simulink model "Audio_Signal_Processing"  (R2020b)
settings: Solver=FixedStepDiscrete  StartTime=0.0  StopTime=10  RelTol=1e-3
libraries: dsparch4 x3, dspvision x1, audioeffects x1
settings Model: Creator=jferrari  LastModifiedBy=Jack
settings SolverCC: AutoInsertRateTranBlk=on
settings DataIOCC: LimitDataPoints=on  SaveOutput=off  SignalLogging=off  SaveTime=off
settings OptimizationCC: LifeSpan=inf
settings DebuggingCC: AlgebraicLoopMsg=error  SingleTaskRateTransMsg=error  AllowSymbolicDim=off  SFUnexpectedBacktrackingDiag=warning  SFNoUnconditionalDefaultTransitionDiag=warning  SFExecutionAtInitializationDiag=none  ArithmeticOperatorsInVariantConditions=warning
settings SFSimCC: SimUseLocalCustomCode=off  CustomCodeUndefinedFunction=UseInterfaceOnly
settings RTWCC: RTWUseLocalCustomCode=off
settings CodeAppCC: StateflowObjectComments=on
settings GRTTargetCC: TargetLangStandard=C89/C90 (ANSI)
settings ConfigComp: CovMetricSettings=dw  CovSaveCumulativeToWorkspaceVar=on  CovSaveSingleToWorkspaceVar=on  CovExternalEMLEnable=off  CovSFcnEnable=off

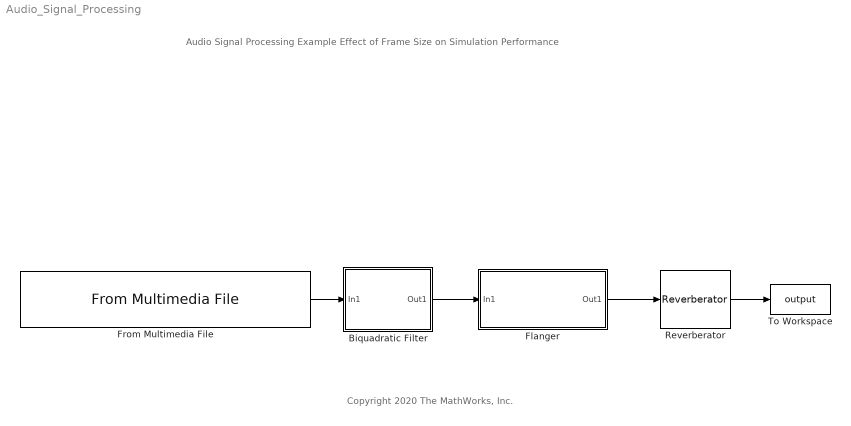
== system Audio_Signal_Processing ==
  note: Copyright 2020 The MathWorks, Inc.
  note: Audio Signal Processing Example
      | Effect of Frame Size on Simulation Performance
  Biquadratic Filter : Subsystem
  Flanger : Subsystem  mask(Flanger){Delay=0.001, Depth=30, Rate=0.25, FeedbackLevel=0.4, WetDryMix=0.5, SampleRate=44100}
      mask prompts: Delay "Base delay (s)"; Rate "Rate (Hz)"; FeedbackLevel "Feedback gain"; WetDryMix "Wet/dry mix"; SampleRate "Input sample rate (Hz):"
      mask help: Apply flanging effect on audio signal.
      mask Display: disp('Flanger')
  From Multimedia File : dspvision/From Multimedia File  inputFilename=/Users/Jack/OneDrive - MathWorks/Documents/Simulink/DSP Project/Frame-Based Processing Example/RockGuitar-16-44p1-stereo-10secs.mp3  readRange=[1 Inf]  loop=on  numPlays=1  outputStreams=Audio only  videoDataType=single  audioDataType=double  inheritSampleTime=on  userDefinedSampleTime=1/30  noAudioOutput=off  isIntensityVideo=off  fourcc=RGB  colorVideoFormat=Separate color signals  outputEOF=off  dataOrg=Column-major  audioFrameSize=1024  computeAudioFrameSize=off  outSamplingMode=Sample based
  Reverberator : audioeffects/Reverberator  PreDelayPort=off  PreDelay=0.0  HighCutFrequencyPort=off  HighCutFrequency=17003.0  DiffusionPort=off  Diffusion=0.0  DecayFactorPort=off  DecayFactor=0.790  HighFrequencyDampingPort=off  HighFrequencyDamping=0.0005  WetDryMixPort=off  WetDryMix=0.3  InheritSampleRate=on  SampleRate=44100  SimulateUsing=Interpreted execution
      settings: SourceProductBaseCode=AU
  To Workspace : ToWorkspace  VariableName=output  SampleTime=-1
      settings: Save2DSignal=2-D array (concatenate along first dimension)
  wires:
  From Multimedia File/1 -> Biquadratic Filter/1(In1)
  Reverberator/1 -> To Workspace/1
  Biquadratic Filter/1(Out1) -> Flanger/1(In1)
  Flanger/1(Out1) -> Reverberator/1

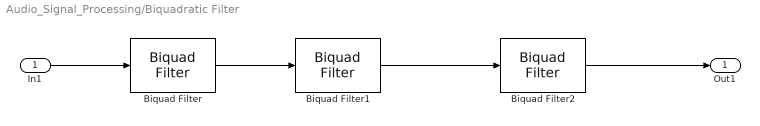
== system Audio_Signal_Processing/Biquadratic Filter ==
  In1 : Inport
  Biquad Filter : dsparch4/Biquad Filter  FilterSource=Dialog parameters  CoeffSource=Specify via dialog  FilterObject=BQF  IIRFiltStruct=Direct form I  BiQuadCoeffs=[1 0.3 0.4 1 0.1 0.2]  ScaleValues=1  IC=0  ICnum=0  ICden=0  a0Flag=Warning  optimizeScaleValues=on  ScaleValueMode=Specify via input port (g)  InputProcessing=Columns as channels (frame based)  roundingMode=Floor  overflowMode=off  scaleValueFracLength=14  denProdOutputFracLength=30  denAccumFracLength=30  secondMemoryFracLength=15
  Biquad Filter1 : dsparch4/Biquad Filter  FilterSource=Dialog parameters  CoeffSource=Specify via dialog  FilterObject=BQF  IIRFiltStruct=Direct form I  BiQuadCoeffs=[1 0.68 -0.4 1 0.4 -0.2]  ScaleValues=1  IC=0  ICnum=0  ICden=0  a0Flag=Warning  optimizeScaleValues=on  ScaleValueMode=Specify via input port (g)  InputProcessing=Columns as channels (frame based)  roundingMode=Floor  overflowMode=off  scaleValueFracLength=14  denProdOutputFracLength=30  denAccumFracLength=30  secondMemoryFracLength=15
  Biquad Filter2 : dsparch4/Biquad Filter  FilterSource=Dialog parameters  CoeffSource=Specify via dialog  FilterObject=BQF  IIRFiltStruct=Direct form I  BiQuadCoeffs=[1 0.62 -0.41 1 0.75 0.2]  ScaleValues=1  IC=0  ICnum=0  ICden=0  a0Flag=Warning  optimizeScaleValues=on  ScaleValueMode=Specify via input port (g)  InputProcessing=Columns as channels (frame based)  roundingMode=Floor  overflowMode=off  scaleValueFracLength=14  denProdOutputFracLength=30  denAccumFracLength=30  secondMemoryFracLength=15
  Out1 : Outport
  wires:
  Biquad Filter/1 -> Biquad Filter1/1
  In1/1 -> Biquad Filter/1
  Biquad Filter1/1 -> Biquad Filter2/1
  Biquad Filter2/1 -> Out1/1

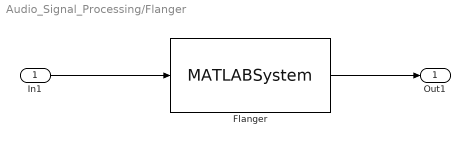
== system Audio_Signal_Processing/Flanger ==
  In1 : Inport
  Flanger : MATLABSystem  System=audioexample.Flanger  Delay=Delay  Depth=Depth  Rate=Rate  FeedbackLevel=FeedbackLevel  WetDryMix=WetDryMix  SampleRate=SampleRate  SimulateUsing=Code generation
      mask Type: audioexample.Flanger
      mask Display:
      | disp('Flanger');
      | port_label('input',1,'Input');
      | port_label('output',1,'Output');
  Out1 : Outport  VectorParamsAs1DForOutWhenUnconnected=off
  wires:
  In1/1 -> Flanger/1
  Flanger/1 -> Out1/1
